simulink library "simulink"  (Simulink 7.6)
settings: Solver=ode45  SolverMode=SingleTasking  StartTime=0.0  StopTime=10.0  RelTol=1e-3
PostLoadFcn:
  | setsysloc(bdroot)
undefined symbols (not defined in the file or in its folder): DiscIntNeverNeededParam, Floor, getdatatypespecs, NumBits1, NumBits2, sfunxy, sigbuilder_block, slcm, SlDemoSign, Slope1, Slope2
libraries: simulink x40, sl_helperblocks x2, eml_lib x1
(part 2 of 5)

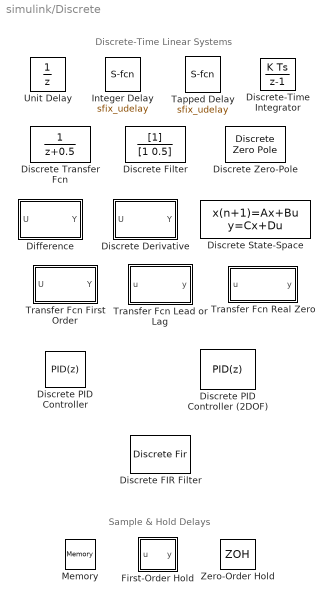
== system simulink/Discrete ==
  note: Sample & Hold Delays
  note: Discrete-Time Linear Systems
  Difference : Subsystem  mask(Difference){ICPrevInput=0.0, OutMin=[], OutMax=[], OutDataTypeStr=Inherit: Inherit via internal rule, OutputDataTypeScalingMode=Inherit via internal rule, OutDataType=fixdt(1, 16), OutScaling=2^-10, LockScale=off, RndMeth=Floor, DoSatur=off}
      mask prompts: ICPrevInput "Initial condition for previous input:"; OutMin "Output minimum:"; OutMax "Output maximum:"; OutDataTypeStr "Output data type:"; OutputDataTypeScalingMode "Output data type mode:"; OutDataType "Output data type (e.g. fixdt(1, 16), fixdt('single')):"; OutScaling "Output scaling (Slope, e.g. 2^-9 or [Slope Bias], e.g. [1.25 3]):"; LockScale "Lock output data type setting against changes by the fixed-point tools"; RndMeth "Integer rounding mode:"; DoSatur "Saturate to max or min when overflows occur"
      mask help: Output the current input value minus the previous input value.
      mask init:
      | blkH = gcbh;
      | blkName = getfullname(blkH);
      | 
      | set_param([blkName,'/Diff'], ...
      |     'RndMeth',RndMeth, ...
      | 	'DoSatur',DoSatur);
      mask StyleString: edit,min,max,unidt({m=4|5|6||7|2|3|}{i=Inherit: Inherit via internal rule|Inherit: Inherit via back propagation}{b=double|single|int8|uint8|int16|uint16|int32|uint32}{s=UDTBinaryPointMode|UDTSlopeBiasMode}{g=UDTSignedSign|UDTUnsignedSign}),popup(double|single|int8|uint8|int16|uint16|int32|uint32|Specify via dialog|Inherit via internal rule|Inherit via back propagation),edit,edit,checkbox,popup(Ceiling|Convergent|Floor|Nearest|Round|Simplest|Zero),checkbox
      mask CallbackString: |||fixptdialog(gcbh)|fixptdialog(gcbh)|fixptdialog(gcbh)||||
      mask TabNameString: Main,Signal Attributes,Signal Attributes,Signal Attributes,Signal Attributes,Signal Attributes,Signal Attributes,Signal Attributes,Signal Attributes,Signal Attributes
      mask Display: dpoly([1 -1],[1 0],'z')
  Discrete Transfer Fcn : DiscreteTransferFcn
  Discrete Zero-Pole : DiscreteZeroPole  Poles=[0 0.5]  Gain=1
  Discrete Derivative : Subsystem  mask(Discrete Derivative){gainval=1.0, ICPrevScaledInput=0.0, OutMin=[], OutMax=[], OutDataTypeStr=Inherit: Inherit via internal rule, OutputDataTypeScalingMode=Inherit via internal rule, OutDataType=fixdt(1, 16), OutScaling=2^-10, LockScale=off, RndMeth=Floor, DoSatur=off}
      mask prompts: gainval "Gain value:"; ICPrevScaledInput "Initial condition for previous weighted input K*u/Ts:"; OutMin "Output minimum:"; OutMax "Output maximum:"; OutDataTypeStr "Output data type:"; OutputDataTypeScalingMode "Output data type mode:"; OutDataType "Output data type (e.g. fixdt(1, 16), fixdt('single')):"; OutScaling "Output scaling (Slope, e.g. 2^-9 or [Slope Bias], e.g. [1.25 3]):"; LockScale "Lock output data type setting against changes by the fixed-point tools"; RndMeth "Integer rounding mode:"; DoSatur "Saturate to max or min when overflows occur"
      mask help:
      | Discrete-time derivative of the input.
      |
      | This block only works with fixed sample rates, so it will not work inside a triggered subsystem.
      mask init:
      | blkH = gcbh;
      | blkName = getfullname(blkH);
      | 
      | if (gainval == 0.0)
      |     %avoid divide by zero warning
      |     inverseGainval = inf;
      | else
      |     inverseGainval = 1.0/double(gainval);
      | end
      | 
      | switch OutputDataTypeScalingMode
      |   case 'Inherit via internal rule'
      |     diffMode   = 'Inherit via back propagation';
      |     tsampMode  = 'Inherit via internal rule';
      |     tsampImp   = 'Offline Scaling Adjustment';
      |   otherwise
      |     diffMode  = OutputDataTypeScalingMode;
      |     tsampMode = 'Inherit via back propagation';
      |     tsampImp  = 'Online Calculations';
      | end
      | if ~strcmp(get_param(bdroot(blkH),'SimulationStatus'), 'running')
      | set_param([blkName,'/Diff'], ...
      |     'OutputDataTypeScalingMode', diffMode, ...
      | 	'RndMeth',RndMeth, ...
      | 	'DoSatur',DoSatur);
      | set_param([blkName,'/TSamp'], ...
      |     'OutputDataTypeScalingMode',tsampMode, ...
      | 	'RndMeth',RndMeth, ...
      | 	'DoSatur',DoSatur, ...
      |     'TsampMathImp',tsampImp);
      | end
      mask StyleString: edit,edit,min,max,unidt({m=5|6|7||8|3|4|}{i=Inherit: Inherit via internal rule|Inherit: Inherit via back propagation}{b=double|single|int8|uint8|int16|uint16|int32|uint32}{s=UDTBinaryPointMode|UDTSlopeBiasMode}{g=UDTSignedSign|UDTUnsignedSign}),popup(double|single|int8|uint8|int16|uint16|int32|uint32|Specify via dialog|Inherit via internal rule|Inherit via back propagation),edit,edit,checkbox,popup(Ceiling|Convergent|Floor|Nearest|Round|Simplest|Zero),checkbox
      mask CallbackString: ||||fixptdialog(gcbh)|fixptdialog(gcbh)|fixptdialog(gcbh)||||
      mask TabNameString: Main,Main,Signal Attributes,Signal Attributes,Signal Attributes,Signal Attributes,Signal Attributes,Signal Attributes,Signal Attributes,Signal Attributes,Signal Attributes
      mask Display: text(0.5, 0.5, 'K (z-1)', 'horizontalAlignment', 'center', 'verticalAlignment', 'bottom');text(0.5, 0.5, 'Ts z', 'horizontalAlignment', 'center', 'verticalAlignment', 'top');plot([0.3 0.7],[0.5 0.5]);
  Discrete FIR Filter : DiscreteFir
  Discrete Filter : DiscreteFilter  SampleTime=1
  Discrete PID Controller : simulink/Continuous/PID Controller  DialogController=pidpack.PIDConfig.pidDDGCreate  DialogControllerArgs=DataTag2  SystemSampleTime=-1  Controller=PID  TimeDomain=Discrete-time  SampleTime=1  IntegratorMethod=Forward Euler  FilterMethod=Forward Euler  Form=Parallel  P=1  I=1  D=0  N=100  InitialConditionSource=internal  InitialConditionForIntegrator=0  InitialConditionForFilter=0  ExternalReset=none  LimitOutput=off  UpperSaturationLimit=inf  LowerSaturationLimit=-inf  LinearizeAsGain=off  AntiWindupMode=none  Kb=1  TrackingMode=off  Kt=1  PParamMin=[]  PParamMax=[]  IParamMin=[]  IParamMax=[]  DParamMin=[]  DParamMax=[]  NParamMin=[]  NParamMax=[]  KbParamMin=[]  KbParamMax=[]  KtParamMin=[]  KtParamMax=[]  POutMin=[]  POutMax=[]  IOutMin=[]  IOutMax=[]  DOutMin=[]  DOutMax=[]  NOutMin=[]  NOutMax=[]  KbOutMin=[]  KbOutMax=[]  KtOutMin=[]  KtOutMax=[]  IntegratorOutMin=[]  IntegratorOutMax=[]  FilterOutMin=[]  FilterOutMax=[]  SumOutMin=[]  SumOutMax=[]  SumI1OutMin=[]  SumI1OutMax=[]  SumI2OutMin=[]  SumI2OutMax=[]  SumI3OutMin=[]  SumI3OutMax=[]  SumDOutMin=[]  SumDOutMax=[]  SaturationOutMin=[]  SaturationOutMax=[]  IntegratorContinuousStateAttributes=''  IntegratorStateMustResolveToSignalObject=off  IntegratorRTWStateStorageClass=Auto  FilterContinuousStateAttributes=''  FilterStateMustResolveToSignalObject=off  FilterRTWStateStorageClass=Auto
  Discrete PID Controller (2DOF) : simulink/Continuous/PID Controller (2DOF)  DialogController=pidpack.PIDConfig.pidDDGCreate  DialogControllerArgs=DataTag3  SystemSampleTime=-1  Controller=PID  TimeDomain=Discrete-time  SampleTime=1  IntegratorMethod=Forward Euler  FilterMethod=Forward Euler  Form=Parallel  P=1  I=1  D=0  N=100  b=1  c=1  InitialConditionSource=internal  InitialConditionForIntegrator=0  InitialConditionForFilter=0  ExternalReset=none  LimitOutput=off  UpperSaturationLimit=inf  LowerSaturationLimit=-inf  LinearizeAsGain=off  AntiWindupMode=none  Kb=1  TrackingMode=off  Kt=1  PParamMin=[]  PParamMax=[]  IParamMin=[]  IParamMax=[]  DParamMin=[]  DParamMax=[]  NParamMin=[]  NParamMax=[]  bParamMin=[]  bParamMax=[]  cParamMin=[]  cParamMax=[]  KbParamMin=[]  KbParamMax=[]  KtParamMin=[]  KtParamMax=[]  POutMin=[]  POutMax=[]  IOutMin=[]  IOutMax=[]  DOutMin=[]  DOutMax=[]  NOutMin=[]  NOutMax=[]  bOutMin=[]  bOutMax=[]  cOutMin=[]  cOutMax=[]  KbOutMin=[]  KbOutMax=[]  KtOutMin=[]  KtOutMax=[]  IntegratorOutMin=[]  IntegratorOutMax=[]  FilterOutMin=[]  FilterOutMax=[]  SumOutMin=[]  SumOutMax=[]  Sum1OutMin=[]  Sum1OutMax=[]  Sum2OutMin=[]  Sum2OutMax=[]  Sum3OutMin=[]  Sum3OutMax=[]  SumI1OutMin=[]  SumI1OutMax=[]  SumI2OutMin=[]  SumI2OutMax=[]  SumI3OutMin=[]  SumI3OutMax=[]  SumDOutMin=[]  SumDOutMax=[]  SaturationOutMin=[]  SaturationOutMax=[]  IntegratorContinuousStateAttributes=''  IntegratorStateMustResolveToSignalObject=off  IntegratorRTWStateStorageClass=Auto  FilterContinuousStateAttributes=''  FilterStateMustResolveToSignalObject=off  FilterRTWStateStorageClass=Auto
  Discrete State-Space : DiscreteStateSpace
  Discrete-Time Integrator : DiscreteIntegrator  ICPrevOutput=DiscIntNeverNeededParam  ICPrevScaledInput=DiscIntNeverNeededParam
  First-Order Hold : Subsystem  DisableCoverage=on  mask(First-Order Hold){Ts=1}
      mask prompts: Ts "Sample time:"
      mask help: First-order hold.
      mask Help: This block implements a first-order hold by extrapolating between sample points using a first-order polynomial.
      mask Display: plot(0,0,100,100,[90,70,50,30,10],[60,40,80,30,20])
  Integer Delay : S-Function  FunctionName=sfix_udelay  Parameters=samptime,vinit,NumDelays,1,1,0,InputProcessing  EnableBusSupport=off  mask(Integer Delay){NumDelays=4, InputProcessing=Elements as channels (sample based), vinit=0.0, samptime=-1}
      mask prompts: NumDelays "Number of delays:"; InputProcessing "Input processing:"; vinit "Initial condition:"; samptime "Sample time:"
      mask help: Delay a signal N sample periods.
      mask init:
      | if isempty(NumDelays)
      |    NumDelays = 1;
      | end
      | slSetFrameUpgradeParameter(gcbh,'InputProcessing','Inherited');
      mask StyleString: edit,popup(Columns as channels (frame based)|Elements as channels (sample based)|Inherited),edit,edit
      mask Display: fprintf(' %d\nZ   ',-1*(NumDelays))
  Memory : Memory
  Tapped Delay : S-Function  FunctionName=sfix_udelay  Parameters=samptime,vinit,NumDelays,NumDelays,DelayOrder,includeCurrent,3  EnableBusSupport=off  mask(Tapped Delay Line){vinit=0.0, samptime=-1, NumDelays=4, DelayOrder=Oldest, includeCurrent=off}
      mask prompts: vinit "Initial condition:"; samptime "Sample time:"; NumDelays "Number of delays:"; DelayOrder "Order output vector starting with:"; includeCurrent "Include current input in output vector"
      mask help: Delay a signal N sample periods and output all the delay versions.
      mask init:
      | if isempty(NumDelays)
      |    NumDelays = 1;
      | end
      mask StyleString: edit,edit,edit,popup(Oldest|Newest),checkbox
      mask Display: fprintf(' %d\nDelays\n',(NumDelays))
  Transfer Fcn First Order : Subsystem  mask(First Order Transfer Fcn){PoleZ=0.95, ICPrevOutput=0.0, RndMeth=Floor, DoSatur=off}
      mask prompts: PoleZ "Pole (in Z plane):"; ICPrevOutput "Initial condition for previous output:"; RndMeth "Integer rounding mode:"; DoSatur "Saturate to max or min when overflows occur"
      mask help: Discrete-time first order transfer function. The transfer function has a unity DC gain.
      mask init:
      | blkH = gcbh;
      | blkName = getfullname(blkH);
      | 
      | vRndMeth = get_param(blkH,'RndMeth');
      | vDoSatur = get_param(blkH,'DoSatur');
      | 
      | set_param([blkName,'/Gain'],'RndMeth',vRndMeth, ...
      | 	'DoSatur',vDoSatur);
      | set_param([blkName,'/Diff'],'RndMeth',vRndMeth, ...
      | 	'DoSatur',vDoSatur);
      | set_param([blkName,'/Sum'],'RndMeth',vRndMeth, ...
      | 	'DoSatur',vDoSatur);
      mask StyleString: edit,edit,popup(Ceiling|Convergent|Floor|Nearest|Round|Simplest|Zero),checkbox
      mask Display: dpoly([1-PoleZ 0],[1 -PoleZ],'z')
  Transfer Fcn Lead or Lag : Subsystem  mask(Lead or Lag Compensator){PoleZ=0.95, ZeroZ=0.75, ICPrevOutput=0.0, ICPrevInput=0.0, RndMeth=Floor, DoSatur=off}
      mask prompts: PoleZ "Pole of compensator (in Z plane):"; ZeroZ "Zero of compensator (in Z plane):"; ICPrevOutput "Initial condition for previous output:"; ICPrevInput "Initial condition for previous input:"; RndMeth "Integer rounding mode:"; DoSatur "Saturate to max or min when overflows occur"
      mask help:
      | Discrete-time lead or lag compensator.  The compensator has a unity instantaneous gain, the DC gain equals (1-Zero)/(1-Pole).
      |
      | Lead compensation is obtained when 0 < Pole < Zero < 1.
      | Lag compensation is obtained when 0 < Zero < Pole < 1.
      mask init:
      | if ((PoleZ < 0) || (PoleZ >= 1))
      |    error('Pole position must be a positive number less than 1')
      | end
      | if ((ZeroZ < 0) || (ZeroZ > 1))
      |    error('Zero position must be a positive number less than or equal to 1')
      | end
      | blkH = gcbh;
      | blkName = getfullname(blkH);
      | 
      | vRndMeth = get_param(blkH,'RndMeth');
      | vDoSatur = get_param(blkH,'DoSatur');
      | DCGain = (1-ZeroZ)./(1-PoleZ);
      | maxGain = max( 1, max(max(abs(DCGain))) );
      | OutputSlopeMult = 2^ceil(log2(maxGain));
      | set_param([blkName,'/GainZero'],'RndMeth',vRndMeth, ...
      | 	'DoSatur',vDoSatur);
      | set_param([blkName,'/GainPole'],'RndMeth',vRndMeth, ...
      | 	'DoSatur',vDoSatur);
      | set_param([blkName,'/Downcast'],'RndMeth',vRndMeth, ...
      | 	'DoSatur',vDoSatur);
      | set_param([blkName,'/Sum'],'RndMeth',vRndMeth, ...
      | 	'DoSatur',vDoSatur);
      mask StyleString: edit,edit,edit,edit,popup(Ceiling|Convergent|Floor|Nearest|Round|Simplest|Zero),checkbox
      mask Display: dpoly([1 -ZeroZ],[1 -PoleZ],'z')
  Transfer Fcn Real Zero : Subsystem  mask(Transfer Fcn Real Zero){ZeroZ=0.75, ICPrevInput=0.0, RndMeth=Floor, DoSatur=off}
      mask prompts: ZeroZ "Zero (in Z plane):"; ICPrevInput "Initial condition for previous input:"; RndMeth "Integer rounding mode:"; DoSatur "Saturate to max or min when overflows occur"
      mask help: Discrete-time transfer function that has a real zero and (effectively) has no pole.
      mask init:
      | blkH = gcbh;
      | blkName = getfullname(blkH);
      | 
      | vRndMeth = get_param(blkH,'RndMeth');
      | vDoSatur = get_param(blkH,'DoSatur');
      | DCGain = (1-ZeroZ);
      | maxGain = max( 1, max(max(abs(DCGain))) );
      | OutputSlopeMult = 2^ceil(log2(maxGain));
      | set_param([blkName,'/GainZero'],'RndMeth',vRndMeth, ...
      | 	'DoSatur',vDoSatur);
      | set_param([blkName,'/Sum'],'RndMeth',vRndMeth, ...
      | 	'DoSatur',vDoSatur);
      mask StyleString: edit,edit,popup(Ceiling|Convergent|Floor|Nearest|Round|Simplest|Zero),checkbox
      mask Display: dpoly([1 -ZeroZ],[1 0],'z')
  Unit Delay : UnitDelay  SampleTime=-1
  Zero-Order Hold : ZeroOrderHold

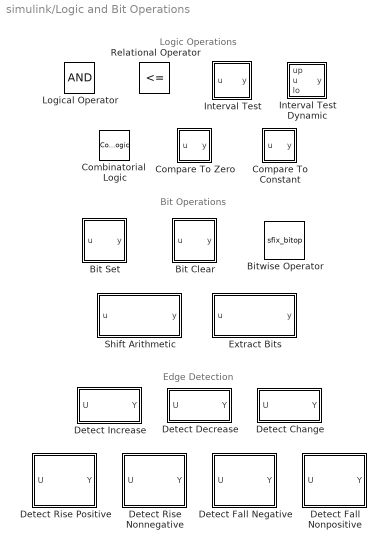
== system simulink/Logic and Bit Operations ==
  note: Edge Detection
  note: Logic Operations
  note: Bit Operations
  Bit Clear : Subsystem  mask(Bit Clear){iBit=0}
      mask prompts: iBit "Index of bit (0 is least significant):"
      mask help: Clear ith bit of the stored integer to 0. Scaling is ignored.
      mask init:
      | if length(iBit) == 1
      |   dispStr = sprintf('Clear\nbit %d',double(iBit));
      | else
      |   dispStr=sprintf('Vector\nBit Clear');
      | end
      mask Display: disp(dispStr)
  Bit Set : Subsystem  mask(Bit Set){iBit=0}
      mask prompts: iBit "Index of bit (0 is least significant):"
      mask help: Set ith bit of the stored integer to 1. Scaling is ignored.
      mask init:
      | if length(iBit) == 1
      |   dispStr = sprintf('Set\nbit %d',double(iBit));
      | else
      |   dispStr=sprintf('Vector\nBit Set');
      | end
      mask Display: disp(dispStr)
  Bitwise Operator : S-Function  FunctionName=sfix_bitop  Parameters=UseBitMask,NumInputPorts,BitMask,BitMaskRealWorld,logicop  EnableBusSupport=off  mask(Bitwise Operator){logicop=AND, UseBitMask=on, NumInputPorts=1, BitMask=bin2dec('11011001'), BitMaskRealWorld=Stored Integer}
      mask prompts: logicop "Operator:"; UseBitMask "Use bit mask ..."; NumInputPorts "Number of input ports:"; BitMask "Bit Mask"; BitMaskRealWorld "Treat mask as:"
      mask help: Perform the specified bitwise operation on the inputs. The output data type should represent zero exactly.
      mask init:
      | str = '';
      | if UseBitMask
      |   [m,n] = size(BitMask);
      |   if ischar(BitMask)
      |     len = m;
      |     n = 1;
      |   else
      |     len = m * n;
      |   end
      |   internalBitMask = zeros(m,n);
      |   if isnumeric(BitMask)
      |     for i=1:len,
      |       internalBitMask(i) = BitMask(i);
      |     end
      |   elseif ischar(BitMask)
      |     for i=1:m,
      |       internalBitMask(i) = hex2dec(BitMask(i,:));
      |     end
      |   elseif iscell(BitMask)
      |     for i=1:len,
      |       if isnumeric( BitMask{i} )
      |         internalBitMask(i) = BitMask{i};
      |       elseif ischar( BitMask{i} )
      |         internalBitMask(i) = hex2dec(BitMask{i});
      |       else
      |         errordlg(['Data type is not supported at cell item ', num2str(i) ]);
      |       end
      |     end
      |   end
      |   BitMask = internalBitMask;
      |   for i=1:len
      |     if BitMask(i) > (2^52)-1
      |       error(DAStudio.message('Simulink:blocks:BitMaskWordLengthTooLarge')); 
      |     end
      |   end 
      |   if len == 1
      |      if BitMaskRealWorld == 1 || BitMask(1) < 0
      |        str=num2str(BitMask(1));
      |      else
      |        str=['0x',dec2hex(floor(BitMask(1)))];
      |      end
      |   else
      |      str='Masks';
      |   end
      | else
      |   BitMask = 0;
      |   str='';
      | end
      mask StyleString: popup(AND|OR|NAND|NOR|XOR|NOT),checkbox,edit,edit,popup(Real World Value|Stored Integer)
      mask CallbackString: fixptdialog(gcbh)|fixptdialog(gcbh)|||
      mask Display: fprintf(['Bitwise\n',logicop,'\n',str])
  Combinatorial  Logic : CombinatorialLogic
  Compare To Constant : Subsystem  mask(Compare To Constant){relop=<=, const=3.0, LogicOutDataTypeMode=uint8, ZeroCross=on}
      mask prompts: relop "Operator:"; const "Constant value:"; LogicOutDataTypeMode "Output data type mode:"; ZeroCross "Enable zero-crossing detection"
      mask help: Determine how a signal compares to a constant.
      mask init:
      | blkName = gcb;
      | 
      | if strcmp(get_param(gcbh,'LogicOutDataTypeMode'),'boolean')
      | 	setValue = 'Boolean';
      | else
      | 	setValue = 'Specify via dialog';
      | end
      | 
      | set_param([blkName,'/Compare'],'relop',relop, ...
      | 	'LogicOutDataTypeMode', setValue, 'ZeroCross', ZeroCross);
      | 
      | str = [relop,' C']; %default
      | 
      | const_str = get_param(blkName, 'const');
      | 
      | if isempty(strfind(const_str, ' ')) && isempty(strfind(const_str, ','))
      |     % scalar or single expression
      |     if isempty(str2num(const_str))
      |         %expression
      |         str = [relop, ' ', const_str];
      |     elseif length(const) == 1
      |         str = [relop,' ',num2str(double(const))];
      |     end
      | end
      mask StyleString: popup(==|~=|<|<=|>=|>),edit,popup(uint8|boolean),checkbox
      mask CallbackString: |||sl('zeroCrossEnable', gcbh);
      mask Display: disp(str)
  Compare To Zero : Subsystem  mask(Compare To Zero){relop=<=, LogicOutDataTypeMode=uint8, ZeroCross=on}
      mask prompts: relop "Operator:"; LogicOutDataTypeMode "Output data type mode:"; ZeroCross "Enable zero-crossing detection"
      mask help: Determine how a signal compares to zero.
      mask init:
      | blkName = gcb;
      | 
      | if strcmp(get_param(gcbh,'LogicOutDataTypeMode'),'boolean')
      | 	setValue = 'Boolean';
      | else
      |     setValue = 'Specify via dialog';
      | end
      | 
      | set_param([blkName,'/Compare'],'relop',relop, ...
      | 	'LogicOutDataTypeMode', setValue, 'ZeroCross', ZeroCross);
      mask StyleString: popup(==|~=|<|<=|>=|>),popup(uint8|boolean),checkbox
      mask CallbackString: ||sl('zeroCrossEnable', gcbh);
      mask Display: disp([relop,' 0'])
  Detect Change : Subsystem  mask(Detect Change){vinit=0}
      mask prompts: vinit "Initial condition:"
      mask help: If the input does not equal its previous value, then output TRUE, otherwise output FALSE. The initial condition determines the initial value of the previous input U/z.
      mask Display: fprintf('U ~= U/z')
  Detect Decrease : Subsystem  mask(Detect Decrease){vinit=0.0}
      mask prompts: vinit "Initial condition:"
      mask help: If the input is strictly less than its previous value, then output TRUE, otherwise output FALSE. The initial condition determines the initial value of the previous input U/z.
      mask Display: fprintf('U < U/z')
  Detect Increase : Subsystem  mask(Detect Increase){vinit=0.0}
      mask prompts: vinit "Initial condition:"
      mask help: If the input is strictly greater than its previous value, then output TRUE, otherwise output FALSE. The initial condition determines the initial value of the previous input U/z.
      mask Display: fprintf('U > U/z')
  Detect Fall Negative : Subsystem  mask(Detect Fall Negative){vinit=0}
      mask prompts: vinit "Initial condition:"
      mask help: If the input is strictly negative and its previous value was nonnegative, then output TRUE, otherwise output FALSE. The initial condition determines the initial value of the boolean expression (U/z < 0).
      mask init:
      | vinit=double(vinit);
      mask Display: fprintf('U < 0\n&  NOT\nU/z < 0')
  Detect Fall Nonpositive : Subsystem  mask(Detect Fall Nonpositive){vinit=0}
      mask prompts: vinit "Initial condition:"
      mask help: If the input is nonpositive and its previous value was strictly positive, then output TRUE, otherwise output FALSE. The initial condition determines the initial value of the boolean expression (U/z <= 0).
      mask init:
      | vinit=double(vinit);
      mask Display: fprintf('U <= 0\n&  NOT\nU/z <= 0')
  Detect Rise Nonnegative : Subsystem  mask(Detect Rise Nonnegative){vinit=0}
      mask prompts: vinit "Initial condition:"
      mask help: If the input is nonnegative and its previous value was strictly negative, then output TRUE, otherwise output FALSE. The initial condition determines the initial value of the boolean expression (U/z >= 0).
      mask init:
      | vinit=double(vinit);
      mask Display: fprintf('U >= 0\n&  NOT\nU/z >= 0')
  Detect Rise Positive : Subsystem  mask(Detect Rise Positive){vinit=0}
      mask prompts: vinit "Initial condition:"
      mask help: If the input is strictly positive and its previous value was nonpositive, then output TRUE, otherwise output FALSE. The initial condition determines the initial value of the boolean expression (U/z > 0).
      mask init:
      | vinit=double(vinit);
      mask Display: fprintf('U > 0\n&  NOT\nU/z > 0')
  Extract Bits : Subsystem  mask(Extract Bits){bitsToExtract=Upper half, numBits=8, bitIdxRange=[0 7], outScalingMode=Preserve fixed-point scaling}
      mask prompts: bitsToExtract "Bits to extract:"; numBits "Number of bits:"; bitIdxRange "Bit indices ([start end], 0-based relative to LSB):"; outScalingMode "Output scaling mode:"
      mask help: Output selected bits from each of the fixed-point input samples. Selecting "Upper half" or "Lower half" results in a positive number of bits in the output word length, according to the equation numOutputBits = ceil(numInputBits / 2).
      mask init:
      | str = fixpt_extractbits_mask('icon', numBits, bitIdxRange); 
      | fixpt_extractbits_mask_script;
      mask StyleString: popup(Upper half|Lower half|Range starting with most significant bit|Range ending with least significant bit|Range of bits),edit,edit,popup(Preserve fixed-point scaling|Treat bit field as an integer)
      mask CallbackString: fixpt_extractbits_mask;|||
      mask Display: disp(str);
  Interval Test : Subsystem  mask(Interval Test){IntervalClosedRight=on, uplimit=0.5, IntervalClosedLeft=on, lowlimit=-0.5, LogicOutDataTypeMode=boolean}
      mask prompts: IntervalClosedRight "Interval closed on right"; uplimit "Upper limit:"; IntervalClosedLeft "Interval closed on left"; lowlimit "Lower limit:"; LogicOutDataTypeMode "Output data type mode:"
      mask help: If the input is in the interval between the lower limit and the upper limit, then the output is TRUE, otherwise it is FALSE.
      mask init:
      | if IntervalClosedLeft
      |   lOff = 0;
      |   lRelop = '<=';
      | else
      |   lOff = 0.1;
      |   lRelop = '<';
      | end
      | if IntervalClosedRight
      |   rOff = 0;
      |   uRelop = '<=';
      | else
      |   rOff = 0.1;
      |   uRelop = '<';
      | end
      | 
      | blkH = gcbh;
      | blkName = getfullname(blkH);
      | 
      | set_param([blkName,'/Upper Test'],'relop',uRelop);
      | set_param([blkName,'/Lower Test'],'relop',lRelop);
      | if strcmp(get_param(blkH,'LogicOutDataTypeMode'),'boolean')
      | set_param([blkName,'/AND'],'OutDataTypeMode','Boolean');
      | else
      | set_param([blkName,'/AND'],'OutDataTypeMode','Specify via dialog');
      | end
      mask StyleString: checkbox,edit,checkbox,edit,popup(uint8|boolean)
      mask Display: plot([0 1],[0.3 0.3],[0.3 0.3],[0 1],[0 0.2 0.2],[0.35 0.35 0.55-lOff],[0.2 0.2 0.55 0.55],[0.55+lOff 0.75 0.75 0.55+rOff],[0.55 0.55 1],[0.55-rOff 0.35 0.35]);
  Interval Test Dynamic : Subsystem  mask(Interval Test Dynamic){IntervalClosedRight=on, IntervalClosedLeft=on, LogicOutDataTypeMode=boolean}
      mask prompts: IntervalClosedRight "Interval closed on right"; IntervalClosedLeft "Interval closed on left"; LogicOutDataTypeMode "Output data type mode:"
      mask help: If the input is in the interval between the lower limit and the upper limit, then the output is TRUE, otherwise it is FALSE.
      mask init:
      | if IntervalClosedLeft
      |   lOff = 0;
      |   lRelop = '<=';
      | else
      |   lOff = 0.1;
      |   lRelop = '<';
      | end
      | if IntervalClosedRight
      |   rOff = 0;
      |   uRelop = '<=';
      | else
      |   rOff = 0.1;
      |   uRelop = '<';
      | end
      | blkH = gcbh;
      | blkName = getfullname(gcbh);
      | 
      | set_param([blkName,'/Upper Test'],'relop',uRelop);
      | set_param([blkName,'/Lower Test'],'relop',lRelop);
      | if strcmp(get_param(blkH,'LogicOutDataTypeMode'),'boolean')
      | set_param([blkName,'/FixPt Logical Operator'],'OutDataTypeMode','Boolean');
      | else
      | set_param([blkName,'/FixPt Logical Operator'],'OutDataTypeMode','Specify via dialog');
      | end
      mask StyleString: checkbox,checkbox,popup(uint8|boolean)
      mask Display: plot(0.35+0.65*[0 1],[0.3 0.3],0.35+0.65*[0.3 0.3],[0 1],0.35+0.65*[0 0.2 0.2],[0.35 0.35 0.55-lOff],0.35+0.65*[0.2 0.2 0.55 0.55],[0.55+lOff 0.75 0.75 0.55+rOff],0.35+0.65*[0.55 0.55 1],[0.55-rOff 0.35 0.35]);
  Logical Operator : Logic  AllPortsSameDT=off  OutDataTypeStr=boolean
  Relational Operator : RelationalOperator  Operator=<=  OutDataTypeStr=boolean
  Shift Arithmetic : Subsystem  mask(Shift Arithmetic){nBitShiftRight=8, nBinPtShiftRight=0}
      mask prompts: nBitShiftRight "Number of bits to shift right (use negative value to shift left):"; nBinPtShiftRight "Number of places by which binary point shifts right (use negative value to shift left):"
      mask help:
      | This block can arithmetically shift the bits and/or the binary point of a signal.
      | The effect of these actions can be interpreted as a combination of a multiplication by a power of two and a change in scaling.  The power of two multiplication term is
      |   2^( NumBinaryPointShiftsRight - NumBitShiftsRight )
      | Negative values for shifts right are actually positive shift lefts.
      | If the input is a floating point type, the power of two multiplication is carried out, but no change in scaling is applied.
      mask init:
      | netExponent = nBinPtShiftRight - nBitShiftRight;
      | netExponent(find(netExponent>127)) = 127;
      | netExponent(find(netExponent<-127)) = -127;
      | nBitShiftRight(find(nBitShiftRight>127)) = 127;
      | nBitShiftRight(find(nBitShiftRight<-127)) = -127;
      | dstr = ['Vy = Vu'];
      | if netExponent ~= 0
      |   dstr = [dstr,' * 2^',num2str(netExponent)];
      | end
      | dstr = [dstr,'\nQy = Qu'];
      | if nBitShiftRight > 0
      |   dstr = [dstr,' >> ',num2str(nBitShiftRight)];
      | elseif nBitShiftRight < 0
      |  dstr = [dstr,' << ',num2str(-nBitShiftRight)];
      | end
      | dstr = [dstr,'\nEy = Eu'];
      | if nBinPtShiftRight > 0
      |   dstr = [dstr,' + ',num2str(nBinPtShiftRight)];
      | elseif nBinPtShiftRight < 0
      |   dstr = [dstr,' - ',num2str(-nBinPtShiftRight)];
      | end
      | for i = 1:length(netExponent)
      |     netExponent(i) = 2^netExponent(i);
      | end
      mask Display: fprintf(dstr)

== system simulink/Lookup Tables ==
  note: Lookup Tables
  Cosine : Subsystem  mask(Sine and Cosine){Formula=cos(2*pi*u), NumDataPoints=(2^5)+1, OutputWordLength=16}
      mask prompts: Formula "Output formula"; NumDataPoints "Number of data points for lookup table:"; OutputWordLength "Output word length:"
      mask help:
      | Implement sine and cosine functions in fixed point using a lookup table approach that exploits quarter wave symmetry. The output fraction length equals the output word length minus 2.
      |
      | The most efficient implementation is obtained when the number of data points is (2^n)+1 where n is an integer.
      mask init:
      | if (~isnumeric(OutputWordLength)) || ( length(OutputWordLength) > 1 ) || ( OutputWordLength < 2 ) || ( floor(OutputWordLength) ~= OutputWordLength )
      |     error(DAStudio.message('Simulink:blocks:SineLookupWordLengthTooSmall'));
      | end
      | if (~isnumeric(NumDataPoints)) || ( length(NumDataPoints) > 1 ) || ( NumDataPoints < 2 ) || ( floor(NumDataPoints) ~= NumDataPoints )
      |     error(DAStudio.message('Simulink:blocks:SineLookupNumDataPtsTooSmall'));
      | end
      | if ( 2^(OutputWordLength-2) + 1 ) < NumDataPoints
      |     smallEnoughNumDataPoints = ( 2^(OutputWordLength-2) + 1 );
      |     bigEnoughOutputWordLength = ceil(log2(NumDataPoints-1))+2;
      |     error(DAStudio.message('Simulink:blocks:SineLookupEitherTooSmall',...
      |         NumDataPoints, ...
      |         smallEnoughNumDataPoints, ...
      |         OutputWordLength, ...
      |         bigEnoughOutputWordLength));
      | end
      | slsincos(Formula);
      mask StyleString: popup(sin(2*pi*u)|cos(2*pi*u)|exp(j*2*pi*u)|sin(2*pi*u) and cos(2*pi*u)),edit,edit
  Direct Lookup Table (n-D) : LookupNDDirect
  Interpolation Using Prelookup : Interpolation_n-D
  Lookup Table Dynamic : S-Function  FunctionName=sfix_look1_dyn  Parameters=OutputDataTypeScalingMode,(getdatatypespecs(OutDataType,OutScaling,DblOver,0, 0, OutputDataTypeScalingMode)),[DoSatur RndMeth-1],DblOver,dolog,LookUpMeth  EnableBusSupport=off  mask(Lookup Table Dynamic){LookUpMeth=Interpolation-Use End Values, OutDataTypeStr=fixdt('double'), OutputDataTypeScalingMode=Specify via dialog, OutDataType=fixdt('double'), OutScaling=2^-10, LockScale=off, RndMeth=Floor, DoSatur=off}
      mask prompts: LookUpMeth "Lookup Method:"; OutDataTypeStr "Output data type:"; OutputDataTypeScalingMode "Output data type mode:"; OutDataType "Output data type (e.g. fixdt(1, 16), fixdt('single')):"; OutScaling "Output scaling (Slope, e.g. 2^-9 or [Slope Bias], e.g. [1.25 3]):"; LockScale "Lock output data type setting against changes by the fixed-point tools"; RndMeth "Integer rounding mode:"; DoSatur "Saturate to max or min when overflows occur"
      mask help: Approximate a one-dimensional function using a selected lookup method.
      mask init:
      | DblOver = 0;
      | dolog = 0;
      mask StyleString: popup(Interpolation-Extrapolation|Interpolation-Use End Values|Use Input Nearest|Use Input Below|Use Input Above),unidt({m=2|3|4||5|||}{i=Inherit: Inherit via back propagation}{b=double|single|int8|uint8|int16|uint16|int32|uint32|boolean}{s=UDTBinaryPointMode|UDTSlopeBiasMode}{g=UDTSignedSign|UDTUnsignedSign}),popup(Specify via dialog|Inherit via back propagation),edit,edit,checkbox,popup(Ceiling|Convergent|Floor|Nearest|Round|Simplest|Zero),checkbox
      mask CallbackString: |fixptdialog(gcbh)|fixptdialog(gcbh)|fixptdialog(gcbh)||||
      mask TabNameString: Main,Signal Attributes,Signal Attributes,Signal Attributes,Signal Attributes,Signal Attributes,Signal Attributes,Signal Attributes
      mask Display:
      | port_label('Input',1,'x');
      | port_label('Input',2,'xdat');
      | port_label('Input',3,'ydat');
      | port_label('Output',1,'y');
  Lookup Table (2-D) : Lookup2D  RowIndex=[1:3]  ColumnIndex=[1:3]  Table=[4 5 6;16 19 20;10 18 23]
  Lookup Table (n-D) : Lookup_n-D  InputSameDT=on
  Lookup Table : Lookup  InputValues=[-5:5]  Table=tanh([-5:5])
  Prelookup : PreLookup  BreakpointsData=[10:10:110]  ProcessOutOfRangeInput=Linear extrapolation
  Sine : Subsystem  mask(Sine and Cosine){Formula=sin(2*pi*u), NumDataPoints=(2^5)+1, OutputWordLength=16}
      mask prompts: Formula "Output formula"; NumDataPoints "Number of data points for lookup table:"; OutputWordLength "Output word length:"
      mask help:
      | Implement sine and cosine functions in fixed point using a lookup table approach that exploits quarter wave symmetry. The output fraction length equals the output word length minus 2.
      |
      | The most efficient implementation is obtained when the number of data points is (2^n)+1 where n is an integer.
      mask init: same as simulink/Lookup Tables/Cosine
      mask StyleString: popup(sin(2*pi*u)|cos(2*pi*u)|exp(j*2*pi*u)|sin(2*pi*u) and cos(2*pi*u)),edit,edit
  wires:
  Prelookup/1 -> Interpolation Using Prelookup/1
  Prelookup/2 -> Interpolation Using Prelookup/2

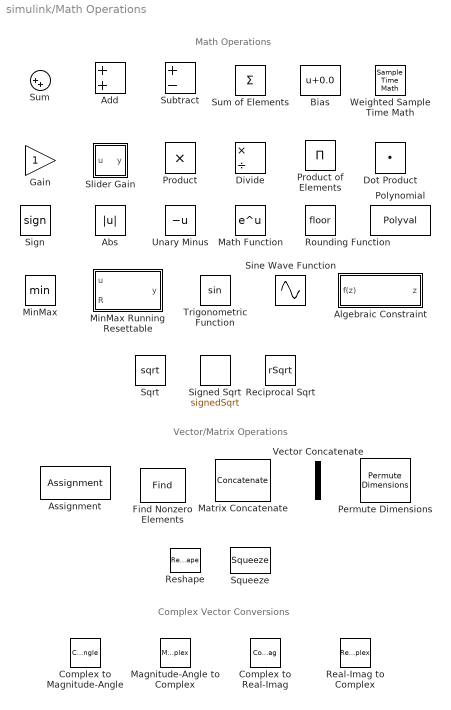
== system simulink/Math Operations ==
  note: Vector/Matrix Operations
  note: Math Operations
  note: Complex Vector Conversions
  Abs : Abs
  Add : Sum
  Algebraic Constraint : Subsystem  mask(Algebraic Constraint){z0=0}
      mask prompts: z0 "Initial guess:"
      mask help: Constrains input signal f(z) to zero and outputs an algebraic state z. This block outputs the value necessary to produce a zero at the input. The output must affect the input through some feedback path. Provide an initial guess of the output to improve algebraic loop solver efficiency.
      mask Help:
      | This block outputs the value necessary to produce a zero at the input. The output must affect the input through some feedback path. This allows you to specify algebraic equations for index 1 differential/algebraic systems (DAE's).
      | 
      | By default, the initial guess is zero.  You can improve the efficiency of the algebraic loop solver by providing an initial guess that is close to the solution value.
      mask Display: disp('Solve\nf(z) = 0')
  Assignment : Assignment  IndexOptions=Index vector (dialog)  Indices=1  OutputSizes=1
  Bias : Bias  Bias=0.0
  Complex to Magnitude-Angle : ComplexToMagnitudeAngle
  Complex to Real-Imag : ComplexToRealImag
  Divide : Product  Inputs=*/
  Dot Product : DotProduct  InputSameDT=on  OutDataTypeStr=Inherit: Inherit via internal rule
  Find Nonzero Elements : Find  NumberOfInputDimensions=3  IndexMode=Zero-based
  Gain : Gain
  Magnitude-Angle to Complex : MagnitudeAngleToComplex
  Math Function : Math  SaturateOnIntegerOverflow=on
  Matrix Concatenate : Concatenate  Mode=Multidimensional array  ConcatenateDimension=2
  MinMax : MinMax
  MinMax Running Resettable : Subsystem  mask(MinMax Running Resettable){Function=min, vinit=0.0}
      mask prompts: vinit "Initial condition:"
      mask help: Output the max or min of all past inputs u. The output is reset to the initial condition when the Reset input signal R is TRUE. This reset action is vectorized and supports scalar expansion.
      mask init:
      | dim = size(vinit);
      | if (length(dim) > 2) || (min(dim) ~= 1)
      |     error('The parameter ''Initial condition'' must be a vector or a scalar');
      |     return;
      | else
      |    set_param([gcb,'/MinMax'],'Function',get_param(gcbh,'Function'));
      | end
      mask StyleString: popup(min|max),edit
      mask Display: disp([char((Function==1)*'min'+(Function==2)*'max'),'(u,y)'])
  Permute Dimensions : PermuteDimensions
  Polynomial : Polyval  Coefs=[ +2.081618890e-019, -1.441693666e-014, +4.719686976e-010, -8.536869453e-006, +1.621573104e-001, -8.087801117e+001 ]
  Product : Product  RndMeth=Zero
  Product of Elements : Product  Inputs=*
  Real-Imag to Complex : RealImagToComplex
  Reciprocal Sqrt : Sqrt  Operator=rSqrt  SaturateOnIntegerOverflow=on
  Reshape : Reshape
  Rounding Function : Rounding
  Sign : Signum
  Signed Sqrt : Sqrt  Operator=signedSqrt  SaturateOnIntegerOverflow=on
  Sine Wave Function : Sin  TimeSource=Use external signal  SampleTime=0
  Slider Gain : Subsystem  LoadFcn=slideg Load  StartFcn=slideg StartFcn  StopFcn=slideg StopFcn  mask(Slider Gain){low=0, gain=1, high=2}
      settings: CopyFcn=slideg Copy  DeleteFcn=slideg DeleteBlock  NameChangeFcn=slideg NameChange  OpenFcn=slideg Open  CloseFcn=slideg Close  ParentCloseFcn=slideg ParentClose
      mask Display: disp(gain)
  Sqrt : Sqrt  SaturateOnIntegerOverflow=on
  Squeeze : Squeeze
  Subtract : Sum  Inputs=+-
  Sum : Sum  Inputs=|++
      settings: CopyFcn=set_param(gcbh,'ShowName','off','CopyFcn','')
  Sum of Elements : Sum  Inputs=+
  Trigonometric Function : Trigonometry
  Unary Minus : UnaryMinus
  Vector Concatenate : Concatenate  Mode=Vector
  Weighted Sample Time Math : SampleTimeMath

== system simulink/Model Verification ==
  note: Run-time Model Verification
  Assertion : Assertion  Enabled=on
  Check Discrete Gradient : Subsystem  Description=| du / dt | < 1  mask(Checks_Gradient){gradient=1, enabled=on, callback=, stopWhenAssertionFail=on, export=off, icon=graphic}
      mask prompts: gradient "Maximum gradient:"; enabled "Enable assertion"; callback "Simulation callback when assertion fails (optional):"; stopWhenAssertionFail "Stop simulation when assertion fails"; export "Output assertion signal"; icon "Select icon type:"
      mask help: Assert that the absolute value of the difference between successive samples of a discrete signal is less than an upper bound.
      mask init:
      | update_assert_sys(gcbh);
      mask StyleString: edit,checkbox,edit,checkbox,checkbox,popup(graphic|text)
      mask CallbackString: |update_assert_sys(gcbh,'updateSimulationCallBackEditField');||||
      mask Display: image(imread('Checks_Gradient.bmp','bmp'),'center')
  Check  Dynamic Gap : Subsystem  Description=sig < min || max < sig  mask(Checks_DGap){enabled=on, callback=, stopWhenAssertionFail=on, export=off, icon=graphic}
      mask prompts: enabled "Enable assertion"; callback "Simulation callback when assertion fails (optional):"; stopWhenAssertionFail "Stop simulation when assertion fails"; export "Output assertion signal"; icon "Select icon type:"
      mask help: Assert that the input signal 'sig' is always less than the lower bound 'min' or greater than the upper bound 'max'. The first input is the upper-bound of the gap; the second input, the lower-bound; the third input, the test signal.
      mask init:
      | update_assert_sys(gcbh);
      mask StyleString: checkbox,edit,checkbox,checkbox,popup(graphic|text)
      mask CallbackString: update_assert_sys(gcbh,'updateSimulationCallBackEditField');||||
      mask Display:
      | port_label('input', 1, 'max');
      | port_label('input', 2, 'min');
      | port_label('input', 3, 'sig');
      | image(imread('Checks_DGap.bmp','bmp'),'center')
  Check  Dynamic Range : Subsystem  Description=min < sig < max  mask(Checks_DRange){enabled=on, callback=, stopWhenAssertionFail=on, export=off, icon=graphic}
      mask prompts: enabled "Enable assertion"; callback "Simulation callback when assertion fails (optional):"; stopWhenAssertionFail "Stop simulation when assertion fails"; export "Output assertion signal"; icon "Select icon type:"
      mask help: Assert that one signal always lies between two other signals. The first input is the upper-bound signal; the second input, the lower-bound; the third input, the test signal.
      mask init:
      | update_assert_sys(gcbh);
      mask StyleString: checkbox,edit,checkbox,checkbox,popup(graphic|text)
      mask CallbackString: update_assert_sys(gcbh,'updateSimulationCallBackEditField');||||
      mask Display:
      | port_label('input', 1,'max');
      | port_label('input', 2, 'min');
      | port_label('input', 3, 'sig');
      | image(imread('Checks_DRange.bmp','bmp'),'center')
  Check  Static Gap : Subsystem  Description=u <= 0 || 100 <= u  mask(Checks_SGap){max=100, max_included=on, min=0, min_included=on, enabled=on, callback=, stopWhenAssertionFail=on, export=off, icon=graphic}
      mask prompts: max "Upper bound:"; max_included "Inclusive upper bound"; min "Lower bound:"; min_included "Inclusive lower bound"; enabled "Enable assertion"; callback "Simulation callback when assertion fails (optional):"; stopWhenAssertionFail "Stop simulation when assertion fails"; export "Output assertion signal"; icon "Select icon type:"
      mask help: Assert that the input signal is less than (or optionally equal to) a static lower bound or greater than (or optionally equal to) a static upper bound.
      mask init:
      | update_assert_sys(gcbh);
      mask StyleString: edit,checkbox,edit,checkbox,checkbox,edit,checkbox,checkbox,popup(graphic|text)
      mask CallbackString: ||||update_assert_sys(gcbh,'updateSimulationCallBackEditField');||||
      mask Display: image(imread('Checks_SGap.bmp','bmp'),'center')
  Check  Static Range : Subsystem  Description=0 <= u <= 100  mask(Checks_SRange){max=100, max_included=on, min=0, min_included=on, enabled=on, callback=, stopWhenAssertionFail=on, export=off, icon=graphic}
      mask prompts: max "Upper bound:"; max_included "Inclusive upper bound"; min "Lower bound:"; min_included "Inclusive lower bound"; enabled "Enable assertion"; callback "Simulation callback when assertion fails (optional):"; stopWhenAssertionFail "Stop simulation when assertion fails"; export "Output assertion signal"; icon "Select icon type:"
      mask help: Assert that the input signal lies between a static lower and upper bound or optionally equals either bound.
      mask init:
      | update_assert_sys(gcbh);
      mask StyleString: edit,checkbox,edit,checkbox,checkbox,edit,checkbox,checkbox,popup(graphic|text)
      mask CallbackString: ||||update_assert_sys(gcbh,'updateSimulationCallBackEditField');||||
      mask Display: image(imread('Checks_SRange.bmp','bmp'),'center')
  Check Dynamic  Lower Bound : Subsystem  Description=min < sig  mask(Checks_DMin){Enabled=on, callback=, stopWhenAssertionFail=on, export=off, icon=graphic}
      mask prompts: Enabled "Enable assertion"; callback "Simulation callback when assertion fails (optional):"; stopWhenAssertionFail "Stop simulation when assertion fails"; export "Output assertion signal"; icon "Select icon type:"
      mask help: Assert that one signal is always less than another signal. The first input is the lower-bound signal. The second input is the test signal.
      mask init:
      | update_assert_sys(gcbh);
      mask StyleString: checkbox,edit,checkbox,checkbox,popup(graphic|text)
      mask CallbackString: update_assert_sys(gcbh,'updateSimulationCallBackEditField');||||
      mask Display:
      | port_label('input', 1,'min');
      | port_label('input', 2, 'sig');
      | image(imread('Checks_DMin.bmp','bmp'),'center')
  Check Dynamic  Upper Bound : Subsystem  Description=sig < max  mask(Checks_DMax){enabled=on, callback=, stopWhenAssertionFail=on, export=off, icon=graphic}
      mask prompts: enabled "Enable assertion"; callback "Simulation callback when assertion fails (optional):"; stopWhenAssertionFail "Stop simulation when assertion fails"; export "Output assertion signal"; icon "Select icon type:"
      mask help: Assert that one signal is always greater than another signal. The first input is the upper-bound signal. The second input is the test signal.
      mask init:
      | update_assert_sys(gcbh);
      mask StyleString: checkbox,edit,checkbox,checkbox,popup(graphic|text)
      mask CallbackString: update_assert_sys(gcbh,'updateSimulationCallBackEditField');||||
      mask Display:
      | port_label('input', 1,'max');
      | port_label('input', 2, 'sig');
      | image(imread('Checks_DMax.bmp','bmp'),'center')
  Check Input  Resolution : Subsystem  Description=-Inf < u < +Inf  mask(Checks_Resolution){resolution=1, enabled=on, callback=, stopWhenAssertionFail=on, export=off}
      mask prompts: enabled "Enable assertion"; callback "Simulation callback when assertion fails (optional):"; stopWhenAssertionFail "Stop simulation when assertion fails"; export "Output assertion signal"
      mask help: Assert that the input signal has a specified resolution. If the resolution is a scalar, the input signal must be a multiple of the resolution within a 10e-3 tolerance. If the resolution is a vector, the input signal must equal an element of the resolution vector.
      mask init:
      | update_assert_sys(gcbh, length(resolution));
      mask CallbackString: |update_assert_sys(gcbh,'updateSimulationCallBackEditField');|||
      mask Display: image(imread('Checks_Resolution.bmp','bmp'),'center')
  Check Static  Lower Bound : Subsystem  Description=0 <= u  mask(Checks_SMin){min=0, min_included=on, enabled=on, callback=, stopWhenAssertionFail=on, export=off, icon=graphic}
      mask prompts: min "Lower bound:"; min_included "Inclusive boundary"; enabled "Enable assertion"; callback "Simulation callback when assertion fails (optional):"; stopWhenAssertionFail "Stop simulation when assertion fails"; export "Output assertion signal"; icon "Select icon type:"
      mask help: Assert that the input signal is greater than (or optionally equal to) a static lower bound.
      mask init:
      | update_assert_sys(gcbh);
      mask StyleString: edit,checkbox,checkbox,edit,checkbox,checkbox,popup(graphic|text)
      mask CallbackString: ||update_assert_sys(gcbh, 'updateSimulationCallBackEditField');||||
      mask Display: image(imread('Checks_SMin.bmp','bmp'),'center')
  Check Static  Upper Bound : Subsystem  Description=u <= 0  mask(Checks_SMax){max=0, max_included=on, enabled=on, callback=, stopWhenAssertionFail=on, export=off, icon=graphic}
      mask prompts: max "Upper bound:"; max_included "Inclusive boundary"; enabled "Enable assertion"; callback "Simulation callback when assertion fails (optional):"; stopWhenAssertionFail "Stop simulation when assertion fails"; export "Output assertion signal"; icon "Select icon type:"
      mask help: Assert that the input signal is less than (or optionally equal to) a static upper bound.
      mask init:
      | update_assert_sys(gcbh);
      mask StyleString: edit,checkbox,checkbox,edit,checkbox,checkbox,popup(graphic|text)
      mask CallbackString: ||update_assert_sys(gcbh,'updateSimulationCallBackEditField');||||
      mask Display: image(imread('Checks_SMax.bmp','bmp'),'center')
